simulink model "dspprogfirhdl"  (Simulink 8.3)
settings: Solver=FixedStepDiscrete  SolverMode=SingleTasking  StartTime=0.0  StopTime=500  RelTol=1e-3
InitFcn:
  | Fpass = 0.45; % Passband Frequency
  | Fstop = 0.55; % Stopband Frequency
  | Apass = 1;    % Passband Attenuation (dB)
  | Astop = 60;   % Stopband Attenuation (dB)
  | 
  | f = fdesign.lowpass('Fp,Fst,Ap,Ast',Fpass,Fstop,Apass,Astop);
  | Hlp = design(f, 'equiripple','FilterStructure', 'dffir'); % Lowpass
  | 
  | Hhp = firlp2hp(Hlp);  % Highpass
  | 
  | Numerator1 = Hlp.Numerator;  % coefficients of lowpass filter
  | Numerator2 = Hhp.Numerator; % coefficients of highpass filter
  | 
  | NTaps = length(Numerator1); % number of coefficients
  | 
  | T = 200; % number of test samples for each set of coefficients
undefined symbols (not defined in the file or in its folder): chirp
libraries: simulink x6, dspmisc x1, dspsrcs4 x1
settings Model: Creator=The MathWorks Inc.
settings DataIOCC: SignalLoggingSaveFormat=Dataset  SaveOutput=off  SaveTime=off  SignalLoggingName=dspprogfirhdl_logsout
settings OptimizationCC: BlockReduction=off  ConditionallyExecuteInputs=off  InlineParams=on  ExpressionDepthLimit=2147483647
settings DebuggingCC: AlgebraicLoopMsg=error  SingleTaskRateTransMsg=error  IntegerOverflowMsg=none  ParameterPrecisionLossMsg=none  FcnCallInpInsideContextMsg=EnableAllAsWarning
settings HardwareCC: ProdHWDeviceType=ASIC/FPGA->ASIC/FPGA  ProdEqTarget=off

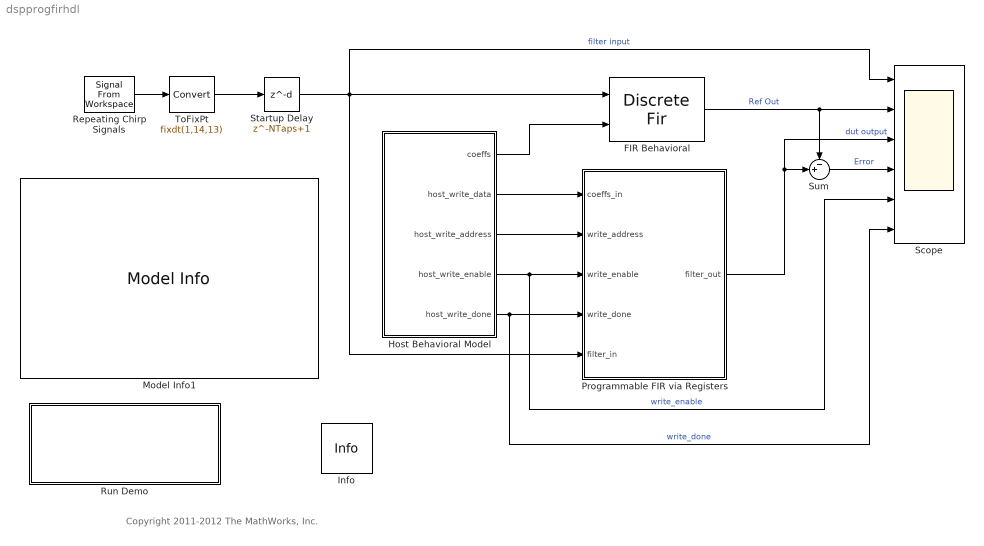
== system dspprogfirhdl ==
  note: Copyright 2011-2012 The MathWorks, Inc.
  FIR Behavioral : DiscreteFir  CoefSource=Input port  Coefficients=Numerator2  InputProcessing=Columns as channels (frame based)  CoefDataTypeStr=fixdt(1,14,13)  ProductDataTypeStr=fixdt(1,29,29)  AccumDataTypeStr=fixdt(1,31,29)  OutDataTypeStr=fixdt(1,14,13)
  Host Behavioral Model : Subsystem
  Info : dspmisc/Info  SystemSampleTime=-1
  Model Info1 : simulink/Model-Wide Utilities/Model Info  InitialBlockCM=None  BlockCM=None  Frame=on  DisplayStringWithTags=|  HorizontalTextAlignment=Left  LeftAlignmentValue=0.02  SourceBlockDiagram=dspprogfirhdl  TagMaxNumber=20
      | Progammable FIR Filter
      | 
      | This model shows a FIR filter whose
      | coefficients are programmable by the
      | host interface. Select fully or serial
      | architecture implementation for Discrete
      | FIR Filter block in HDL Block Properties.
      | 
      | See the Model Properties InitFcn Callback 
      | function to set the filter coefficients.
  Programmable FIR via Registers : Subsystem
  Repeating Chirp Signals : dspsrcs4/Signal From Workspace  X=[chirp(0:T-1,0,T-1,0.4),chirp(0:T-1,0,T-1,0.4)]  Ts=1  nsamps=1  OutputAfterFinalValue=Setting to zero  ignoreOrWarnInputAndFrameLengths=off
  Run Demo : Subsystem
      settings: OpenFcn=hdldialog(bdroot)
      mask Display: disp('Launch HDL Dialog')
  Scope : Scope  NumInputPorts=6
      settings: TimeRange=500  YMin=-1~-1~-1~-1~0~0  YMax=1~1~1~1~2~2  SaveName=ScopeData2
  Startup Delay : Delay  DelayLength=NTaps+1  InputProcessing=Inherited
  Sum : Sum  Inputs=-+|
  ToFixPt : DataTypeConversion  OutDataTypeStr=fixdt(1,14,13)  RndMeth=Nearest  SaturateOnIntegerOverflow=on
  wires:
  Host Behavioral Model/2(host_write_data) -> Programmable FIR via Registers/1(coeffs_in)
  Host Behavioral Model/3(host_write_address) -> Programmable FIR via Registers/2(write_address)
  Host Behavioral Model/4(host_write_enable) -> Programmable FIR via Registers/3(write_enable), Scope/5  "write_enable"
  Host Behavioral Model/5(host_write_done) -> Programmable FIR via Registers/4(write_done), Scope/6  "write_done"
  Programmable FIR via Registers/1(filter_out) -> Scope/3, Sum/2  "dut output"
  FIR Behavioral/1 -> Scope/2, Sum/1  "Ref Out"
  Repeating Chirp Signals/1 -> ToFixPt/1
  Host Behavioral Model/1(coeffs) -> FIR Behavioral/2
  Startup Delay/1 -> FIR Behavioral/1, Scope/1, Programmable FIR via Registers/5(filter_in)  "filter input"
  ToFixPt/1 -> Startup Delay/1
  Sum/1 -> Scope/4  "Error"

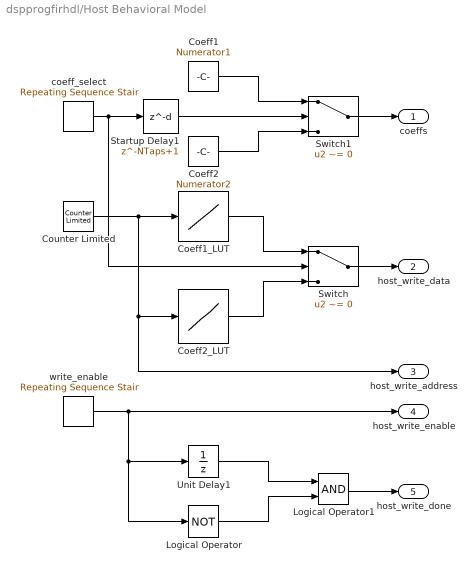
== system dspprogfirhdl/Host Behavioral Model ==
  Coeff1 : Constant  Value=Numerator1  OutDataTypeStr=fixdt(1,14,13)  SampleTime=1
  Coeff1_LUT : Lookup  InputValues=[0:NTaps-1]  Table=Numerator1  LookUpMeth=Use Input Nearest  OutDataTypeStr=fixdt(1,14,13)
  Coeff2 : Constant  Value=Numerator2  OutDataTypeStr=fixdt(1,14,13)  SampleTime=1
  Coeff2_LUT : Lookup  InputValues=[0:NTaps-1]  Table=Numerator2  LookUpMeth=Use Input Nearest  OutDataTypeStr=fixdt(1,14,13)
  Counter Limited : simulink/Sources/Counter Limited  uplimit=NTaps-1  tsamp=-1
  Logical Operator : Logic  Operator=NOT  AllPortsSameDT=off  OutDataTypeStr=boolean
  Logical Operator1 : Logic  AllPortsSameDT=off  OutDataTypeStr=boolean
  Startup Delay1 : Delay  DelayLength=NTaps+1  InputProcessing=Inherited
  Switch : Switch  Criteria=u2 ~= 0
  Switch1 : Switch  Criteria=u2 ~= 0
  Unit Delay1 : UnitDelay  SampleTime=-1
  coeff_select : simulink/Sources/Repeating Sequence Stair  OutValues=[ones(T,1);zeros(T,1)]  tsamp=-1  OutMin=[]  OutMax=[]  OutDataTypeStr=fixdt('boolean')  OutputDataTypeScalingMode=Specify via dialog  OutDataType=fixdt('boolean')  ConRadixGroup=Best Precision: Vector-wise  OutScaling=[]
  write_enable : simulink/Sources/Repeating Sequence Stair  OutValues=[ones(NTaps,1); zeros(T-NTaps,1)]  tsamp=-1  OutMin=[]  OutMax=[]  OutDataTypeStr=fixdt('boolean')  OutputDataTypeScalingMode=Specify via dialog  OutDataType=fixdt('boolean')  ConRadixGroup=Best Precision: Vector-wise  OutScaling=[]
  coeffs : Outport
  host_write_data : Outport  Port=2
  host_write_address : Outport  Port=3
  host_write_enable : Outport  Port=4  OutDataTypeStr=boolean
  host_write_done : Outport  Port=5
  wires:
  Counter Limited/1 -> Coeff1_LUT/1, Coeff2_LUT/1, host_write_address/1
  Coeff1_LUT/1 -> Switch/1
  Switch/1 -> host_write_data/1
  Coeff2_LUT/1 -> Switch/3
  Coeff1/1 -> Switch1/1
  Coeff2/1 -> Switch1/3
  coeff_select/1 -> Startup Delay1/1, Switch/2
  Switch1/1 -> coeffs/1
  Startup Delay1/1 -> Switch1/2
  Unit Delay1/1 -> Logical Operator1/1
  Logical Operator/1 -> Logical Operator1/2
  Logical Operator1/1 -> host_write_done/1
  write_enable/1 -> Logical Operator/1, Unit Delay1/1, host_write_enable/1

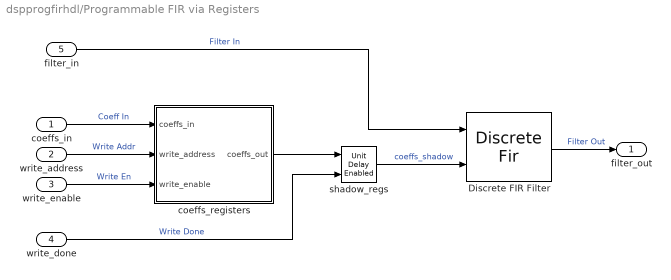
== system dspprogfirhdl/Programmable FIR via Registers ==
  coeffs_in : Inport
  write_address : Inport  Port=2
  write_enable : Inport  Port=3
  write_done : Inport  Port=4
  filter_in : Inport  Port=5  PortDimensions=1
  Discrete FIR Filter : DiscreteFir  CoefSource=Input port  InputProcessing=Columns as channels (frame based)  ProductDataTypeStr=fixdt(1,29,29)  AccumDataTypeStr=fixdt(1,31,29)  OutDataTypeStr=fixdt(1,14,13)
  coeffs_registers : Subsystem  mask(Coefficients registers){numRegs=NTaps}
      mask prompts: numRegs "Number of registers"
      mask help: Store programmable coefficients in a register file, which is writable when 'write_enable' is true.
  shadow_regs : simulink/Additional Math & Discrete/Additional Discrete/Unit Delay Enabled  vinit=0.0  tsamp=-1
  filter_out : Outport
  wires:
  filter_in/1 -> Discrete FIR Filter/1  "Filter In"
  Discrete FIR Filter/1 -> filter_out/1  "Filter Out"
  coeffs_in/1 -> coeffs_registers/1(coeffs_in)  "Coeff In"
  write_address/1 -> coeffs_registers/2(write_address)  "Write Addr"
  write_enable/1 -> coeffs_registers/3(write_enable)  "Write En"
  write_done/1 -> shadow_regs/2  "Write Done"
  coeffs_registers/1(coeffs_out) -> shadow_regs/1
  shadow_regs/1 -> Discrete FIR Filter/2  "coeffs_shadow"

== system dspprogfirhdl/Run Demo ==

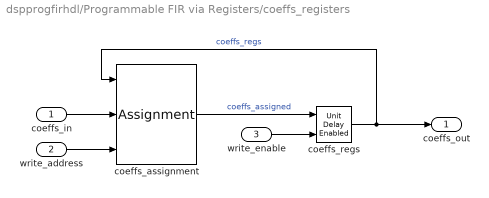
== system dspprogfirhdl/Programmable FIR via Registers/coeffs_registers ==
  coeffs_in : Inport
  write_address : Inport  Port=2
  write_enable : Inport  Port=3
  coeffs_assignment : Assignment  IndexMode=Zero-based  IndexOptions=Index vector (port)  OutputSizes=[1 1]
  coeffs_regs : simulink/Additional Math & Discrete/Additional Discrete/Unit Delay Enabled  vinit=zeros(numRegs,1)  tsamp=-1
  coeffs_out : Outport
  wires:
  coeffs_assignment/1 -> coeffs_regs/1  "coeffs_assigned"
  coeffs_in/1 -> coeffs_assignment/2
  write_enable/1 -> coeffs_regs/2
  write_address/1 -> coeffs_assignment/3
  coeffs_regs/1 -> coeffs_out/1, coeffs_assignment/1  "coeffs_regs"
